simulink model "TestEnvironment"  (R2021b)
settings: Solver=VariableStepAuto  StartTime=0.0  StopTime=50  RelTol=1e-3  EnableMultiTasking=on
libraries: dspsigops x2, simulink_extras x1, simulink x1
settings Model: Creator=ndoehlert  LastModifiedBy=s142
settings SolverCC: AlgebraicLoopSolver=TrustRegion
settings DataIOCC: LimitDataPoints=on  ReturnWorkspaceOutputs=off
settings OptimizationCC: LifeSpan=inf
settings DebuggingCC: AllowSymbolicDim=off  SFUnexpectedBacktrackingDiag=warning  SFNoUnconditionalDefaultTransitionDiag=warning  SFExecutionAtInitializationDiag=none  SFMachineParentedDataDiag=warning  ArithmeticOperatorsInVariantConditions=warning
settings ModelReferenceCC: PropagateSignalLabelsOutOfModel=off
settings SFSimCC: SimUseLocalCustomCode=off  CustomCodeUndefinedFunction=UseInterfaceOnly
settings RTWCC: RTWUseLocalCustomCode=off
settings CodeAppCC: StateflowObjectComments=on
settings GRTTargetCC: TargetLangStandard=C89/C90 (ANSI)
settings ConfigComp: CovMetricSettings=dw  CovSaveCumulativeToWorkspaceVar=on  CovSaveSingleToWorkspaceVar=on  CovExternalEMLEnable=off

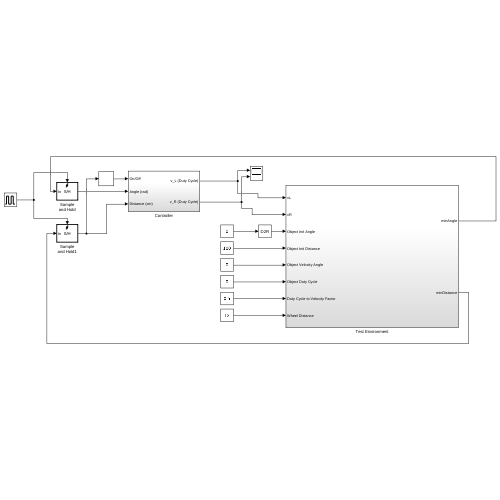
[thumbnail: Simulink's stored preview of the top-level diagram]
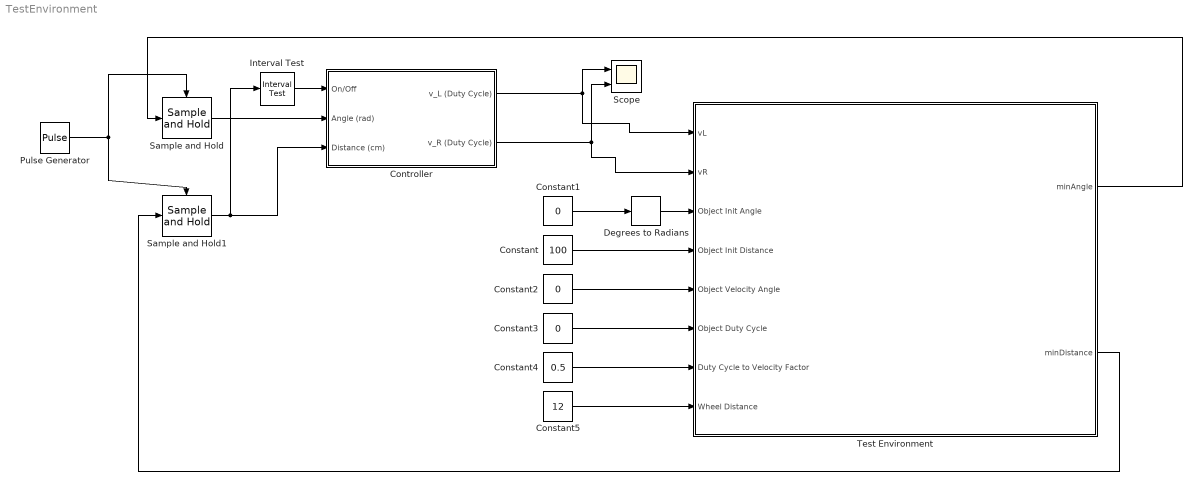
== system TestEnvironment ==
  Constant : Constant  Value=100
  Constant1 : Constant  Value=0
  Constant2 : Constant  Value=0
  Constant3 : Constant  Value=0
  Constant4 : Constant  Value=0.5
  Constant5 : Constant  Value=12
  Controller : Subsystem
  Degrees to Radians : simulink_extras/Transformations/Degrees to Radians
  Interval Test : simulink/Logic and Bit Operations/Interval Test  IntervalClosedRight=on  uplimit=150  IntervalClosedLeft=on  lowlimit=25  OutDataTypeStr=boolean
  Pulse Generator : DiscretePulseGenerator  PulseType=Time based  Period=0.5  PulseWidth=5
  Sample and Hold : dspsigops/Sample and Hold  trig=Rising edge  initCond=0  latchinput=off
  Sample and Hold1 : dspsigops/Sample and Hold  trig=Rising edge  initCond=0  latchinput=off
  Scope : Scope  NumInputPorts=2
  Test Environment : Subsystem
  wires:
  Controller/1(v_L (Duty Cycle)) -> Test Environment/1(vL), Scope/1
  Controller/2(v_R (Duty Cycle)) -> Test Environment/2(vR), Scope/2
  Test Environment/2(minDistance) -> Sample and Hold1/1
  Test Environment/1(minAngle) -> Sample and Hold/1
  Constant/1 -> Test Environment/4(Object Init Distance)
  Constant1/1 -> Degrees to Radians/1
  Degrees to Radians/1 -> Test Environment/3(Object Init Angle)
  Constant2/1 -> Test Environment/5(Object Velocity Angle)
  Constant3/1 -> Test Environment/6(Object Duty Cycle)
  Constant4/1 -> Test Environment/7(Duty Cycle to Velocity Factor)
  Constant5/1 -> Test Environment/8(Wheel Distance)
  Interval Test/1 -> Controller/1(On/Off)
  Sample and Hold/1 -> Controller/2(Angle (rad))
  Sample and Hold1/1 -> Interval Test/1, Controller/3(Distance (cm))
  Pulse Generator/1 -> Sample and Hold/Trigger, Sample and Hold1/Trigger

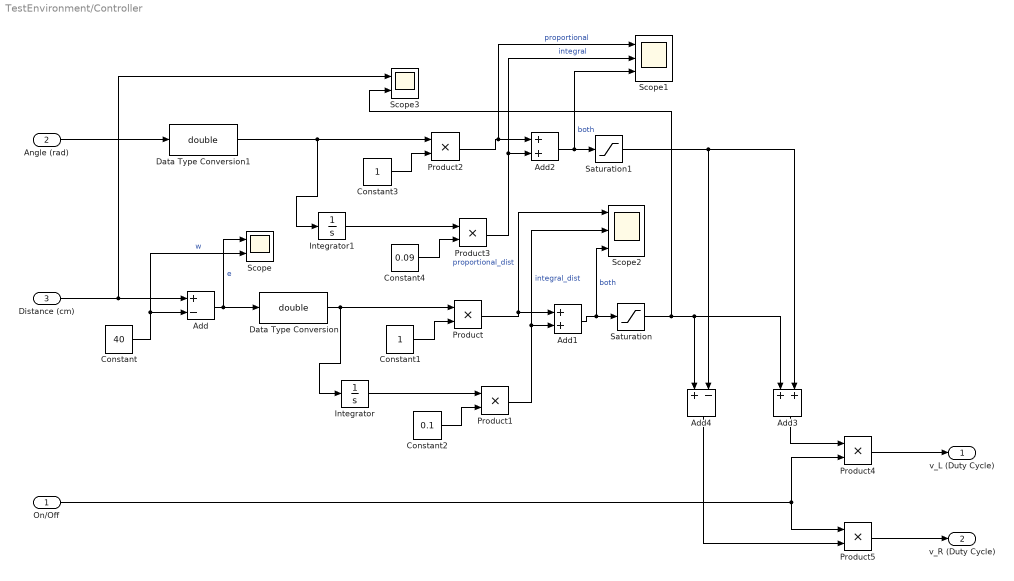
== system TestEnvironment/Controller ==
  On/Off : Inport
  Angle (rad) : Inport  Port=2
  Distance (cm) : Inport  Port=3
  Add : Sum  Inputs=+-
  Add1 : Sum
  Add2 : Sum
  Add3 : Sum
  Add4 : Sum  Inputs=+-
  Constant : Constant  Value=40
  Constant1 : Constant
  Constant2 : Constant  Value=0.1
  Constant3 : Constant
  Constant4 : Constant  Value=0.09
  Data Type Conversion : DataTypeConversion  OutDataTypeStr=double
  Data Type Conversion1 : DataTypeConversion  OutDataTypeStr=double
  Integrator : Integrator
  Integrator1 : Integrator
  Product{,1..5} (6 alike) : Product
  Saturation : Saturate  UpperLimit=100  LowerLimit=-100
  Saturation1 : Saturate  UpperLimit=50  LowerLimit=-50
  Scope : Scope  NumInputPorts=2
  Scope1 : Scope  NumInputPorts=3
  Scope2 : Scope  NumInputPorts=3
  Scope3 : Scope  NumInputPorts=2
  v_L (Duty Cycle) : Outport
  v_R (Duty Cycle) : Outport  Port=2
  wires:
  Add4/1 -> Product5/2
  Product2/1 -> Scope1/1, Add2/1  "proportional"
  Saturation1/1 -> Add4/2, Add3/2
  Data Type Conversion1/1 -> Integrator1/1, Product2/1
  On/Off/1 -> Product5/1, Product4/2
  Angle (rad)/1 -> Data Type Conversion1/1
  Add2/1 -> Scope1/3, Saturation1/1  "both"
  Constant/1 -> Add/2, Scope/2  "w"
  Product1/1 -> Scope2/2, Add1/2  "integral_dist"
  Constant1/1 -> Product/2
  Data Type Conversion/1 -> Integrator/1, Product/1
  Constant3/1 -> Product2/2
  Add1/1 -> Scope2/3, Saturation/1  "both"
  Constant2/1 -> Product1/2
  Distance (cm)/1 -> Scope3/1, Add/1
  Add/1 -> Scope/1, Data Type Conversion/1  "e"
  Integrator1/1 -> Product3/1
  Add3/1 -> Product4/1
  Product3/1 -> Scope1/2, Add2/2  "integral"
  Integrator/1 -> Product1/1
  Constant4/1 -> Product3/2
  Product4/1 -> v_L (Duty Cycle)/1
  Saturation/1 -> Scope3/2, Add3/1, Add4/1
  Product5/1 -> v_R (Duty Cycle)/1
  Product/1 -> Scope2/1, Add1/1  "proportional_dist"

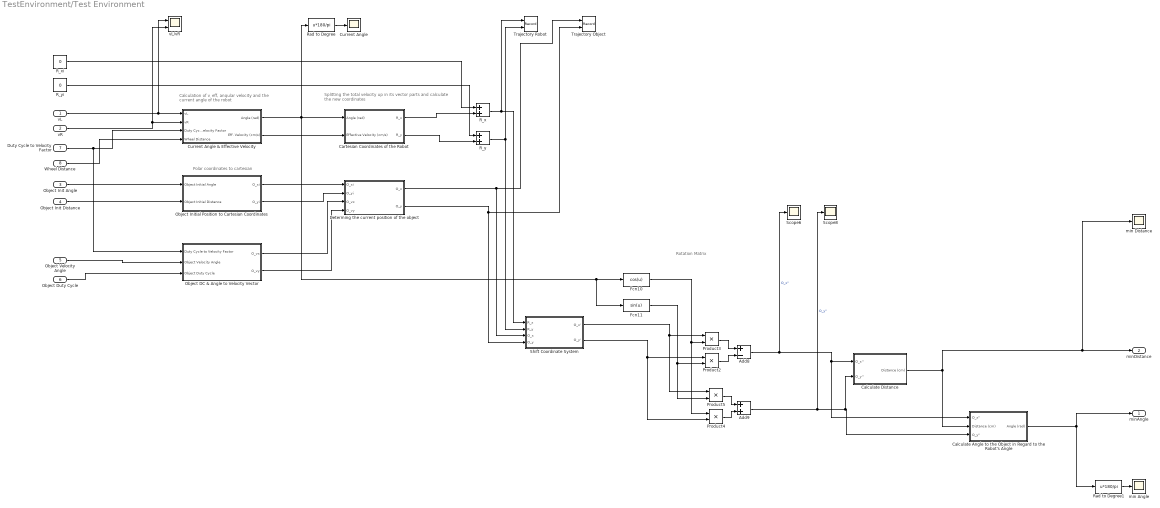
== system TestEnvironment/Test Environment ==
  note: Splitting the total velocity up in its vector parts and calculate
      | the new coordinates
  note: Calculation of v_eff, angular velocity and the
      | current angle of the robot
  note: Rotation Matrix
  note: Polar coordinates to cartesian
  vL : Inport
  vR : Inport  Port=2
  Object Init Angle : Inport  Port=3
  Object Init Distance : Inport  Port=4
  Object Velocity Angle : Inport  Port=5
  Object Duty Cycle : Inport  Port=6
  Duty Cycle to Velocity Factor : Inport  Port=7
  Wheel Distance : Inport  Port=8
  Add8 : Sum  Inputs=+-
  Add9 : Sum
  Calculate Angle to the Object in Regard to the Robot's Angle : Subsystem
  Calculate Distance : Subsystem
  Cartesian Coordinates of the Robot : Subsystem
  Current Angle : Scope
  Current Angle & Effective Velocity : Subsystem
  Determing the current position of the object : Subsystem
  Fcn10 : Fcn  Expr=cos(u)
  Fcn11 : Fcn  Expr=sin(u)
  Object DC & Angle to Velocity Vector : Subsystem
  Object Initial Position to Cartesian Coordinates : Subsystem
  Product{2..5} (4 alike) : Product
  R_x : Sum
  R_xi : Constant  Value=0
  R_y : Sum
  R_yi : Constant  Value=0
  Rad to Degree : Fcn  Expr=u*180/pi
  Rad to Degree1 : Fcn  Expr=u*180/pi
  Scope6 : Scope
  Scope8 : Scope
  Shift Coordinate System : Subsystem
  Trajectory Object : Record  FileSettingsInternal="{\"entries\":[{\"content\":{\"excelSettings\":{\"content\":{},\"type\":\"Streamout.ExcelSettings\"}},\"type\":\"Streamout.FileSettingStorage\",\"uuid\":\"4358cfd4-5c60-4c2b-a41c-9f08c4051154\"}],\"packageUris\":[\"http://schema.mathworks.com/mf0/streamout_blocks/R2020a\"],\"version\":\"1.0\"}"  Layout=[1 1]  SignalsInternal="{\"entries\":[{\"content\":{\"signals\":[{\"content\":{\"blockPath\":[\"TestEnvironment/Test Environment/Trajectory Object\"],\"channel\":[],\"dimensions\":[1],\"domain\":\"TestEnvironment/Test Environment/Trajectory Object\",\"lineColor\":\"#a2142f\",\"plots\":[1],\"port\":1,\"sid\":[\"\"],\"signalID\":97443,\"signalName\":\"Determing the current position of the object:1\"},\"type\":\"RecordBlkView.Signal\",\"uuid\":\"aa5916f7-6d25-42f7-8957-082480ec873f\"},{\"content\":{\"blockPath\":[\"TestEnvironment/Test Environment/Trajectory Object\"],\"channel\":[],\"dimensions\":[1],\"domain\":\"TestEnvironment/Test Environment/Trajectory Object\",\"lineColor\":\"#139fff\",\"plots\":[1],\"port\":2,\"sid\":[\"\"],\"signalID\":97447,\"signalName\":\"Determing the current position of the object:2\"},\"type\":\"RecordBlkView.Signal\",\"uuid\":\"39e0bba6-d15f-46d3-8e29-94819b5ee996\"}]},\"type\":\"RecordBlkView.InputSignals\",\"uuid\":\"a27befac-d0fa-48c7-a9eb-d403d83835f5\"}],\"packageUris\":[\"http://schema.mathworks.com/mf0/streamout_blocks/R2020a\"],\"version\":\"1.0\"}"  VisualizationBindings="{\"xyplotplugin\":{\"info\":[{\"series\":[{\"bindingParametersList\":[{\"parameter\":\"X-Axis\",\"signalID\":97443,\"signalName\":\"Determing the current position of the object:1\"},{\"parameter\":\"Y-Axis\",\"signalID\":97447,\"signalName\":\"Determing the current position of the object:2\"}],\"seriesID\":34098}],\"subplotID\":1}]}}"  CompatibilityTag=XY  st=-1
  Trajectory Robot : Record  FileSettingsInternal="{\"entries\":[{\"content\":{\"excelSettings\":{\"content\":{},\"type\":\"Streamout.ExcelSettings\"}},\"type\":\"Streamout.FileSettingStorage\",\"uuid\":\"ce479cd9-54bd-4dbf-b5c9-76e8a047de80\"}],\"packageUris\":[\"http://schema.mathworks.com/mf0/streamout_blocks/R2020a\"],\"version\":\"1.0\"}"  Layout=[1 1]  SignalsInternal="{\"entries\":[{\"content\":{\"signals\":[{\"content\":{\"blockPath\":[\"TestEnvironment/Test Environment/Trajectory Robot\"],\"channel\":[],\"dimensions\":[1],\"domain\":\"TestEnvironment/Test Environment/Trajectory Robot\",\"lineColor\":\"#a2142f\",\"plots\":[1],\"port\":1,\"sid\":[\"\"],\"signalID\":97451,\"signalName\":\"R_x\"},\"type\":\"RecordBlkView.Signal\",\"uuid\":\"04633b91-b40c-4f09-8643-1ba6794452d3\"},{\"content\":{\"blockPath\":[\"TestEnvironment/Test Environment/Trajectory Robot\"],\"channel\":[],\"dimensions\":[1],\"domain\":\"TestEnvironment/Test Environment/Trajectory Robot\",\"lineColor\":\"#139fff\",\"plots\":[1],\"port\":2,\"sid\":[\"\"],\"signalID\":97455,\"signalName\":\"R_y\"},\"type\":\"RecordBlkView.Signal\",\"uuid\":\"db961c29-ab2a-4748-89ec-817439c60ea6\"}]},\"type\":\"RecordBlkView.InputSignals\",\"uuid\":\"801af185-4798-427f-b3b6-ddf8ac37f784\"}],\"packageUris\":[\"http://schema.mathworks.com/mf0/streamout_blocks/R2020a\"],\"version\":\"1.0\"}"  VisualizationBindings="{\"xyplotplugin\":{\"info\":[{\"series\":[{\"bindingParametersList\":[{\"parameter\":\"X-Axis\",\"signalID\":97451,\"signalName\":\"R_x\"},{\"parameter\":\"Y-Axis\",\"signalID\":97455,\"signalName\":\"R_y\"}],\"seriesID\":34460}],\"subplotID\":1}]}}"  CompatibilityTag=XY  st=-1
  min Angle : Scope
  min Distance : Scope
  vL/vR : Scope  NumInputPorts=2
  minAngle : Outport
  minDistance : Outport  Port=2
  wires:
  vL/1 -> vL/vR/1, Current Angle & Effective Velocity/1(vL)
  vR/1 -> Current Angle & Effective Velocity/2(vR), vL/vR/2
  R_xi/1 -> R_x/1
  R_yi/1 -> R_y/1
  R_x/1 -> Shift Coordinate System/1(R_x), Trajectory Robot/1
  R_y/1 -> Shift Coordinate System/2(R_y), Trajectory Robot/2
  Duty Cycle to Velocity Factor/1 -> Current Angle & Effective Velocity/3(Duty Cycle to Velocity Factor), Object DC & Angle to Velocity Vector/1(Duty Cycle to Velocity Factor)
  Rad to Degree/1 -> Current Angle/1
  Fcn10/1 -> Product4/1, Product3/2
  Fcn11/1 -> Product5/2, Product2/2
  Product3/1 -> Add8/1
  Product2/1 -> Add8/2
  Product5/1 -> Add9/1
  Product4/1 -> Add9/2
  Add8/1 -> Calculate Angle to the Object in Regard to the Robot's Angle/1(O_x''), Calculate Distance/1(O_x''), Scope6/1  "O_x''"
  Add9/1 -> Calculate Distance/2(O_y''), Calculate Angle to the Object in Regard to the Robot's Angle/3(O_y''), Scope8/1  "O_y''"
  Rad to Degree1/1 -> min Angle/1
  Current Angle & Effective Velocity/1(Angle (rad)) -> Fcn11/1, Fcn10/1, Cartesian Coordinates of the Robot/1(Angle (rad)), Rad to Degree/1
  Wheel Distance/1 -> Current Angle & Effective Velocity/4(Wheel Distance)
  Current Angle & Effective Velocity/2(Eff. Velocity (cm/s)) -> Cartesian Coordinates of the Robot/2(Effective Velocity (cm/s))
  Cartesian Coordinates of the Robot/1(R_x) -> R_x/2
  Cartesian Coordinates of the Robot/2(R_y) -> R_y/2
  Object Init Angle/1 -> Object Initial Position to Cartesian Coordinates/1(Object Initial Angle)
  Object Init Distance/1 -> Object Initial Position to Cartesian Coordinates/2(Object Initial Distance)
  Object Velocity Angle/1 -> Object DC & Angle to Velocity Vector/2(Object Velocity Angle)
  Object Duty Cycle/1 -> Object DC & Angle to Velocity Vector/3(Object Duty Cycle)
  Determing the current position of the object/2(O_y) -> Shift Coordinate System/4(O_y), Trajectory Object/2
  Determing the current position of the object/1(O_x) -> Shift Coordinate System/3(O_x), Trajectory Object/1
  Object Initial Position to Cartesian Coordinates/1(O_xi) -> Determing the current position of the object/1(O_xi)
  Object Initial Position to Cartesian Coordinates/2(O_yi) -> Determing the current position of the object/2(O_yi)
  Object DC & Angle to Velocity Vector/1(O_vx) -> Determing the current position of the object/3(O_vx)
  Object DC & Angle to Velocity Vector/2(O_vy) -> Determing the current position of the object/4(O_vy)
  Shift Coordinate System/2(O_y') -> Product4/2, Product2/1
  Shift Coordinate System/1(O_x') -> Product5/1, Product3/1
  Calculate Distance/1(Distance (cm)) -> Calculate Angle to the Object in Regard to the Robot's Angle/2(Distance (cm)), min Distance/1, minDistance/1
  Calculate Angle to the Object in Regard to the Robot's Angle/1(Angle (rad)) -> minAngle/1, Rad to Degree1/1

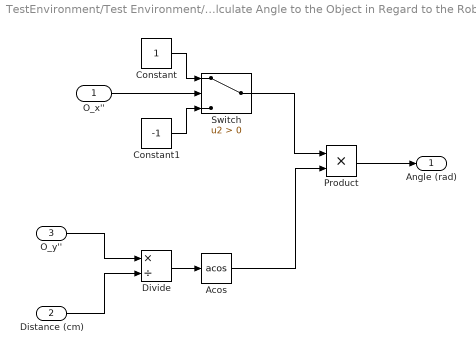
== system TestEnvironment/Test Environment/Calculate Angle to the Object in Regard to the Robot's Angle ==
  O_x'' : Inport
  Distance (cm) : Inport  Port=2
  O_y'' : Inport  Port=3
  Acos : Trigonometry  Operator=acos
  Constant : Constant
  Constant1 : Constant  Value=-1
  Divide : Product  Inputs=*/
  Product : Product
  Switch : Switch  Criteria=u2 > Threshold
  Angle (rad) : Outport
  wires:
  O_x''/1 -> Switch/2
  Constant/1 -> Switch/1
  Constant1/1 -> Switch/3
  O_y''/1 -> Divide/1
  Distance (cm)/1 -> Divide/2
  Divide/1 -> Acos/1
  Acos/1 -> Product/2
  Switch/1 -> Product/1
  Product/1 -> Angle (rad)/1

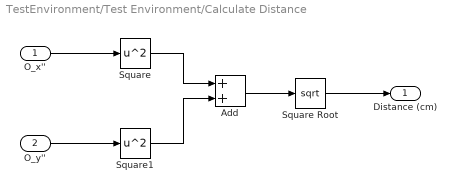
== system TestEnvironment/Test Environment/Calculate Distance ==
  O_x'' : Inport
  O_y'' : Inport  Port=2
  Add : Sum
  Square : Math  Operator=square  SaturateOnIntegerOverflow=on
  Square Root : Sqrt  SaturateOnIntegerOverflow=on
  Square1 : Math  Operator=square  SaturateOnIntegerOverflow=on
  Distance (cm) : Outport
  wires:
  O_y''/1 -> Square1/1
  O_x''/1 -> Square/1
  Square/1 -> Add/1
  Square1/1 -> Add/2
  Add/1 -> Square Root/1
  Square Root/1 -> Distance (cm)/1

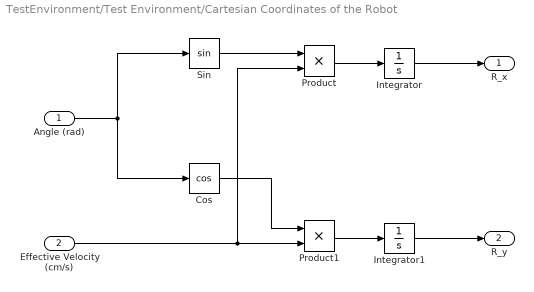
== system TestEnvironment/Test Environment/Cartesian Coordinates of the Robot ==
  Angle (rad) : Inport
  Effective Velocity (cm/s) : Inport  Port=2
  Cos : Trigonometry  Operator=cos
  Integrator : Integrator
  Integrator1 : Integrator
  Product : Product
  Product1 : Product
  Sin : Trigonometry
  R_x : Outport
  R_y : Outport  Port=2
  wires:
  Angle (rad)/1 -> Sin/1, Cos/1
  Sin/1 -> Product/1
  Cos/1 -> Product1/1
  Effective Velocity (cm/s)/1 -> Product/2, Product1/2
  Product/1 -> Integrator/1
  Integrator/1 -> R_x/1
  Product1/1 -> Integrator1/1
  Integrator1/1 -> R_y/1

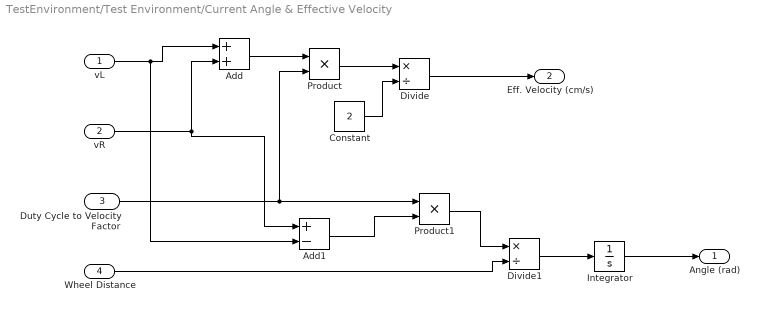
== system TestEnvironment/Test Environment/Current Angle & Effective Velocity ==
  vL : Inport
  vR : Inport  Port=2
  Duty Cycle to Velocity Factor : Inport  Port=3
  Wheel Distance : Inport  Port=4
  Add : Sum
  Add1 : Sum  Inputs=+-
  Constant : Constant  Value=2
  Divide : Product  Inputs=*/
  Divide1 : Product  Inputs=*/
  Integrator : Integrator
  Product : Product
  Product1 : Product
  Angle (rad) : Outport
  Eff. Velocity (cm/s) : Outport  Port=2
  wires:
  vL/1 -> Add1/2, Add/1
  vR/1 -> Add1/1, Add/2
  Add/1 -> Product/1
  Product/1 -> Divide/1
  Constant/1 -> Divide/2
  Divide/1 -> Eff. Velocity (cm/s)/1
  Wheel Distance/1 -> Divide1/2
  Duty Cycle to Velocity Factor/1 -> Product1/1, Product/2
  Product1/1 -> Divide1/1
  Divide1/1 -> Integrator/1
  Integrator/1 -> Angle (rad)/1
  Add1/1 -> Product1/2

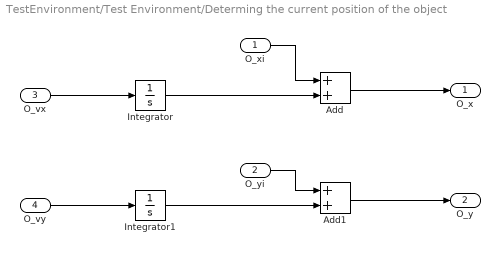
== system TestEnvironment/Test Environment/Determing the current position of the object ==
  O_xi : Inport
  O_yi : Inport  Port=2
  O_vx : Inport  Port=3
  O_vy : Inport  Port=4
  Add : Sum
  Add1 : Sum
  Integrator : Integrator
  Integrator1 : Integrator
  O_x : Outport
  O_y : Outport  Port=2
  wires:
  O_vx/1 -> Integrator/1
  O_vy/1 -> Integrator1/1
  O_xi/1 -> Add/1
  Integrator/1 -> Add/2
  Integrator1/1 -> Add1/2
  O_yi/1 -> Add1/1
  Add/1 -> O_x/1
  Add1/1 -> O_y/1

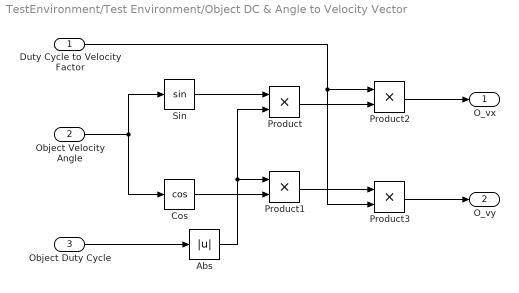
== system TestEnvironment/Test Environment/Object DC & Angle to Velocity Vector ==
  Duty Cycle to Velocity Factor : Inport
  Object Velocity Angle : Inport  Port=2
  Object Duty Cycle : Inport  Port=3
  Abs : Abs
  Cos : Trigonometry  Operator=cos
  Product{,1..3} (4 alike) : Product
  Sin : Trigonometry
  O_vx : Outport
  O_vy : Outport  Port=2
  wires:
  Object Velocity Angle/1 -> Cos/1, Sin/1
  Object Duty Cycle/1 -> Abs/1
  Sin/1 -> Product/1
  Cos/1 -> Product1/2
  Abs/1 -> Product/2, Product1/1
  Product/1 -> Product2/2
  Duty Cycle to Velocity Factor/1 -> Product3/2, Product2/1
  Product1/1 -> Product3/1
  Product2/1 -> O_vx/1
  Product3/1 -> O_vy/1

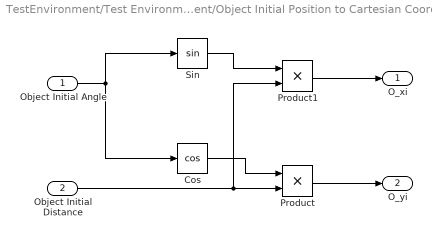
== system TestEnvironment/Test Environment/Object Initial Position to Cartesian Coordinates ==
  Object Initial Angle : Inport
  Object Initial Distance : Inport  Port=2
  Cos : Trigonometry  Operator=cos
  Product : Product
  Product1 : Product
  Sin : Trigonometry
  O_xi : Outport
  O_yi : Outport  Port=2
  wires:
  Object Initial Angle/1 -> Cos/1, Sin/1
  Cos/1 -> Product/1
  Object Initial Distance/1 -> Product1/2, Product/2
  Sin/1 -> Product1/1
  Product1/1 -> O_xi/1
  Product/1 -> O_yi/1

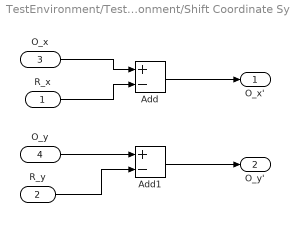
== system TestEnvironment/Test Environment/Shift Coordinate System ==
  R_x : Inport
  R_y : Inport  Port=2
  O_x : Inport  Port=3
  O_y : Inport  Port=4
  Add : Sum  Inputs=+-
  Add1 : Sum  Inputs=+-
  O_x' : Outport
  O_y' : Outport  Port=2
  wires:
  R_x/1 -> Add/2
  O_x/1 -> Add/1
  O_y/1 -> Add1/1
  R_y/1 -> Add1/2
  Add/1 -> O_x'/1
  Add1/1 -> O_y'/1
